simulink model "Car_light"  (R2022a)
settings: Solver=FixedStepAuto  StartTime=0.0  StopTime=100000  FixedStep=1.0  MaxStep=5  RelTol=1e-3
settings Model: DataDictionary=TrafficLightComposer.sldd  Creator=Amin  LastModifiedBy=Amin

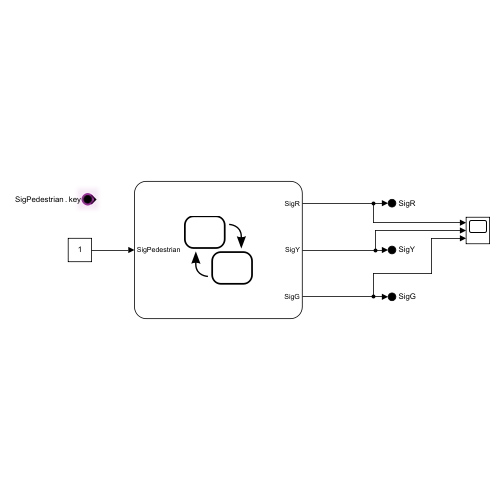
[thumbnail: Simulink's stored preview of the top-level diagram]
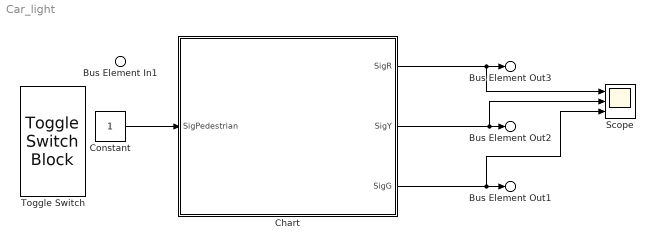
== system Car_light ==
  Bus Element In1 : Inport  PortName=SigPedestrian  Element=key
  Chart : Stateflow chart  TreatAsAtomicUnit=on
  Constant : Constant
  Scope : Scope  NumInputPorts=3
  Toggle Switch : ToggleSwitchBlock
      settings: Values={{'Off', 'On'}, [0 1]}
  Bus Element Out3 : Outport  PortName=SigR
  Bus Element Out2 : Outport  Port=2  PortName=SigY
  Bus Element Out1 : Outport  Port=3  PortName=SigG
  wires:
  Chart/2(SigY) -> Scope/2, Bus Element Out2/1
  Chart/3(SigG) -> Scope/3, Bus Element Out1/1
  Constant/1 -> Chart/1(SigPedestrian)
  Chart/1(SigR) -> Scope/1, Bus Element Out3/1

== stateflow chart Car_light/Chart ==
  state Green
  state Red
  state Pending
  state Yellow
  Green -> Green [order 3] : [count<60]{count=count+1;}
  Green -> Pending [order 1] : [count<60 && SigPedestrian]{count=count+1;}
  Red -> Green [order 1] : [count>=60]{SigG=1;SigR=0;count=0}
  Green -> Yellow [order 2] : [count>=60&&SigPedestrian]{SigY=1;SigG=0;count=0}
  (default) -> Red : {count=0;SigR=1}
  Pending -> Pending [order 2] : {count=count+1;}
  Red -> Red [order 2] : {count=count+1;}
  Yellow -> Red [order 1] : [count>=5]{SigR=1;SigY=0;count=0}
  Pending -> Yellow [order 1] : [count>=60]{SigY=1;SigG=0;count=0;}
  Yellow -> Yellow [order 2] : {count=count+1;}
  data: SigPedestrian input; SigR output; SigY output; SigG output; count local
